simulink model "J1"  (R2019b)
settings: Solver=VariableStepAuto  StartTime=0.0  StopTime=10.0  RelTol=1e-3
values from neighbouring files (symbols this model uses):
  a1 = 0    [bianliang.m]
  a4 = 0    [bianliang.m]
  b11 = 0    [bianliang.m]
  b12 = 0    [bianliang.m]
  b13 = 0    [bianliang.m]
  b4 = 0    [bianliang.m]
  c11 = 0    [bianliang.m]
  c12 = 0    [bianliang.m]
  c13 = 0    [bianliang.m]
  c4 = 0    [bianliang.m]
settings Model: Creator=Inspiron  LastModifiedBy=Inspiron

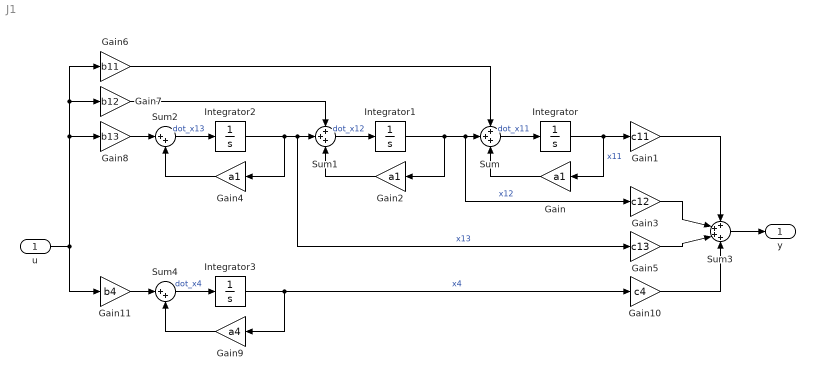
== system J1 ==
  u : Inport
  Gain : Gain  Gain=a1
  Gain1 : Gain  Gain=c11
  Gain10 : Gain  Gain=c4
  Gain11 : Gain  Gain=b4
  Gain2 : Gain  Gain=a1
  Gain3 : Gain  Gain=c12
  Gain4 : Gain  Gain=a1
  Gain5 : Gain  Gain=c13
  Gain6 : Gain  Gain=b11
  Gain7 : Gain  Gain=b12
  Gain8 : Gain  Gain=b13
  Gain9 : Gain  Gain=a4
  Integrator{,1..3} (4 alike) : Integrator
  Sum : Sum  Inputs=+++
  Sum1 : Sum  Inputs=+++
  Sum2 : Sum  Inputs=|++
  Sum3 : Sum  Inputs=++++
  Sum4 : Sum  Inputs=|++
  y : Outport
  wires:
  u/1 -> Gain11/1, Gain6/1, Gain7/1, Gain8/1
  Gain1/1 -> Sum3/1
  Gain3/1 -> Sum3/2
  Gain5/1 -> Sum3/3
  Sum3/1 -> y/1
  Gain7/1 -> Sum1/1
  Gain4/1 -> Sum2/2
  Gain8/1 -> Sum2/1
  Integrator2/1 -> Sum1/2, Gain5/1, Gain4/1  "x13"
  Sum2/1 -> Integrator2/1  "dot_x13"
  Sum1/1 -> Integrator1/1  "dot_x12"
  Integrator1/1 -> Gain3/1, Sum/2, Gain2/1  "x12"
  Integrator/1 -> Gain1/1, Gain/1  "x11"
  Sum/1 -> Integrator/1  "dot_x11"
  Sum4/1 -> Integrator3/1  "dot_x4"
  Gain9/1 -> Sum4/2
  Integrator3/1 -> Gain9/1, Gain10/1  "x4"
  Gain10/1 -> Sum3/4
  Gain/1 -> Sum/3
  Gain2/1 -> Sum1/3
  Gain6/1 -> Sum/1
  Gain11/1 -> Sum4/1
